simulink library "torqueCommand_lib"  (R2022b)
settings: Solver=VariableStepAuto  StartTime=0.0  StopTime=10.0  RelTol=1e-3
undefined symbols (not defined in the file): raptor_xcp_function
libraries: Raptor_lib x3, simulink x1
settings Model: Creator=serga  LastModifiedBy=serga

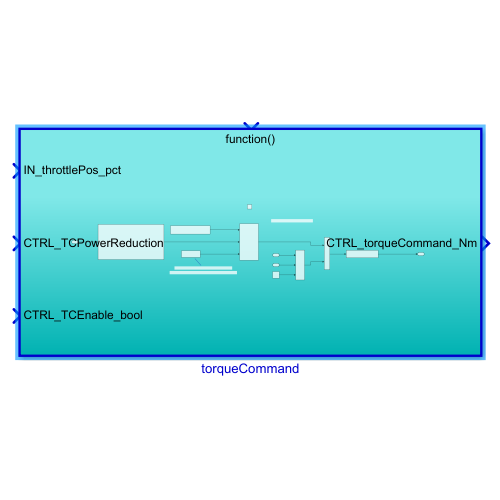
[thumbnail: Simulink's stored preview of the top-level diagram]
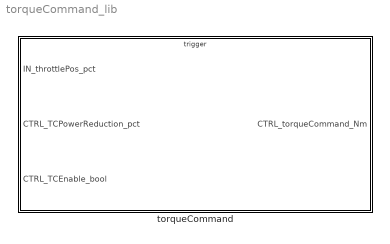
== system torqueCommand_lib ==
  torqueCommand : Subsystem  TreatAsAtomicUnit=on

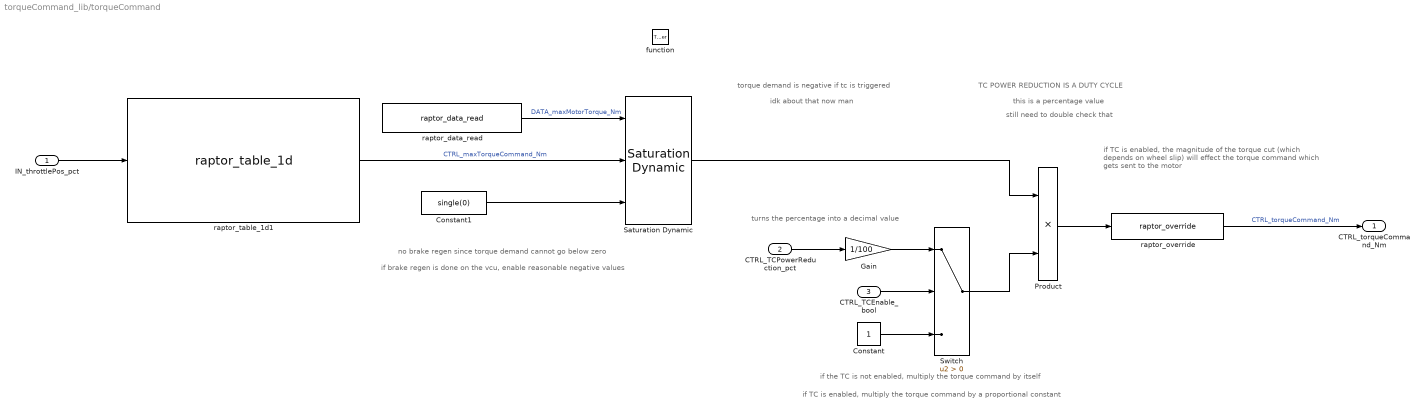
== system torqueCommand_lib/torqueCommand ==
  note: still need to double check that
  note: if TC is enabled, the magnitude of the torque cut (which depends on wheel slip) will effect the torque command which gets sent to the motor
  note: turns the percentage into a decimal value
  note: this is a percentage value
  note: TC POWER REDUCTION IS A DUTY CYCLE
  note: if TC is enabled, multiply the torque command by a proportional constant
  note: if the TC is not enabled, multiply the torque command by itself
  note: idk about that now man
  note: if brake regen is done on the vcu, enable reasonable negative values
  note: no brake regen since torque demand cannot go below zero
  note: torque demand is negative if tc is triggered
  IN_throttlePos_pct : Inport
  CTRL_TCPowerReduction_pct : Inport  Port=2
  CTRL_TCEnable_bool : Inport  Port=3
  function : TriggerPort  TriggerType=function-call  VariantControl=(inherit)
  Constant : Constant
  Constant1 : Constant  Value=single(0)
  Gain : Gain  Gain=1/100
  Product : Product
  Saturation Dynamic : simulink/Discontinuities/Saturation Dynamic  OutMin=[]  OutMax=[]  OutDataTypeStr=Inherit: Same as second input  OutDataType=fixdt(1, 16)  OutScaling=2^-10  DoSatur=off
  Switch : Switch  Criteria=u2 > Threshold  SaturateOnIntegerOverflow=off  InputSameDT=off
  raptor_data_read : Raptor_lib/Data Storage/raptor_data_read  dataName='DATA_maxMotorTorque_Nm'  dataShape=Scalar  idxSource=Input  idxRow=1  idxCol=1
      settings: SourceProductName=Raptor
  raptor_override : Raptor_lib/Data Storage/raptor_override  paramName='DataName'  nameSource=Output Wire  measurement=Output  calDispType=Number  calEnum={'False', 'True'}  calGain=1.0  calOffset=0.0  calMax=inf  calMin=-inf  calFormat='-1'  calUnit=''  calHelp=''  calAccess=1  calFunction="[raptor_xcp_function(gcb) '|'  'Override']"
      settings: SourceProductName=Raptor
  raptor_table_1d1 : Raptor_lib/Table Lookup/raptor_table_1d  dataName='CTRL_throttleToNm'  initValue=[0.0 1.5 3.0 4.5 6.0 7.5 9.0 10.5 12.0 13.5 15.0 16.5 18.0 19.5 21.0 22.5 24.0 25.5 27.0 28.5 30.0 31.5 33.0 34.5 36.0 37.5 39.0 40.5 42.0 43.5 45.0 46.5 48.0 49.5 51.0 52.5 54.0 55.5 57.0 58.5 60.0 61.5 63.0 64.5 66.0 67.5 69.0 70.5 72.0 73.5 75.0 76.5 78.0 79.5 81.0 82.5 84.0 85.5 87.0 88.5 90.0 91.5 93.0 94.5 96.0 97.5 99.0 100.5 102.0 103.5 105.0 106.5 108.0 109.5 111.0 112.5 114.0 115.5 117.0 118.5 120.0]  dataType=single  storage=Calibration  initValueX=|  dataTypeXY=single  storageXY=Calibration  calVisible=on  showTable=on  calGain=1.0  calOffset=0.0  calMax=Inf  calMin=-Inf  calFormat='-1'  calUnit='Nm'  calHelp=''  showBreakpoint=on  dataNameX=[]  calGainX=1.0  calOffsetX=0.0  calMaxX=Inf  calMinX=-Inf  calFormatX='-1'  calUnitX='%'  calHelpX=''  calAccess=1  calFunction=raptor_xcp_function(gcb)  measureEnable=off  mName=['Data1D_Output']
      | [0.0 1.25 2.5 3.75 5.0 6.25 7.5 8.75 10.0 11.25 12.5 13.75 15.0 16.25 17.5 18.75 20.0 21.25 22.5 23.75 25.0 26.25 27.5 28.75 30.0 31.25 32.5 33.75 35.0 36.25 37.5 38.75 40.0 41.25 42.5 43.75 45.0 46.25 47.5 48.75 50.0 51.25 52.5 53.75 55.0 56.25 57.5 58.75 60.0 61.25 62.5 63.75 65.0 66.25 67.5 68.75 70.0 71.25 72.5 73.75 75.0 76.25 77.5 78.75 80.0 81.25 82.5 83.75 85.0 86.25 87.5 88.75 90.0 91.25 92.5 93.75 95.0 96.25 97.5 98.75 100.0
      | ]
      settings: SourceProductName=Raptor
  CTRL_torqueCommand_Nm : Outport
  wires:
  IN_throttlePos_pct/1 -> raptor_table_1d1/1
  Saturation Dynamic/1 -> Product/1
  Constant1/1 -> Saturation Dynamic/3
  raptor_table_1d1/1 -> Saturation Dynamic/2  "CTRL_maxTorqueCommand_Nm"
  raptor_data_read/1 -> Saturation Dynamic/1  "DATA_maxMotorTorque_Nm"
  CTRL_TCEnable_bool/1 -> Switch/2
  CTRL_TCPowerReduction_pct/1 -> Gain/1
  Constant/1 -> Switch/3
  Switch/1 -> Product/2
  Product/1 -> raptor_override/1
  raptor_override/1 -> CTRL_torqueCommand_Nm/1  "CTRL_torqueCommand_Nm"
  Gain/1 -> Switch/1
